simulink model "projeto_final_fm_reduce_freq"  (R2019a)
settings: Solver=ode14x  StartTime=0.0  StopTime=0.59  FixedStep=1e-5  RelTol=1e-3
libraries: dsparch4 x2, commsynccomp2 x1
settings Model: Creator=marco  LastModifiedBy=marco

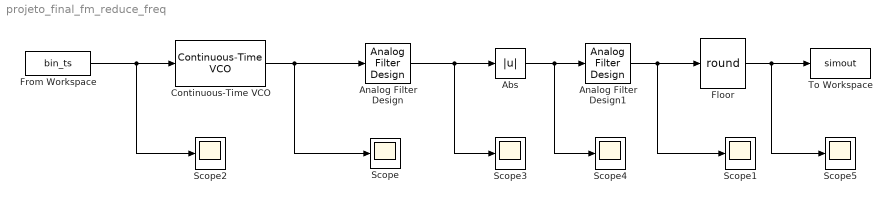
== system projeto_final_fm_reduce_freq ==
  Abs : Abs
  Analog Filter Design : dsparch4/Analog Filter Design  method=Butterworth  filttype=Bandpass  N=8  Wlo=2*pi*(1e4-2.3e3+2.9e3)  Whi=2*pi*(1e4+2.3e3+2.9e3)  Rp=2  Rs=40
  Analog Filter Design1 : dsparch4/Analog Filter Design  method=Butterworth  filttype=Lowpass  N=8  Wlo=2*pi*2e3  Whi=80  Rp=2  Rs=40
  Continuous-Time VCO : commsynccomp2/Continuous-Time VCO  Ac=1  Fc=1e4  Kc=0.1e4  Ph=0
      settings: SourceProductName=Communications Toolbox  SourceProductBaseCode=CM
  Floor : Rounding  Operator=round
  From Workspace : FromWorkspace  VariableName=bin_ts  OutDataTypeStr=double  SampleTime=0  Interpolate=off  OutputAfterFinalValue=Setting to zero
  Scope{,1..5} (6 alike) : Scope
  To Workspace : ToWorkspace  VariableName=simout  SaveFormat=Timeseries  SampleTime=-1
  wires:
  Continuous-Time VCO/1 -> Analog Filter Design/1, Scope/1
  Abs/1 -> Scope4/1, Analog Filter Design1/1
  Analog Filter Design/1 -> Scope3/1, Abs/1
  Analog Filter Design1/1 -> Scope1/1, Floor/1
  From Workspace/1 -> Scope2/1, Continuous-Time VCO/1
  Floor/1 -> Scope5/1, To Workspace/1
